simulink model "state_estimator_opt_driftingcar_multibeta"  (R2017a)
settings: Solver=FixedStepAuto  StartTime=0.0  StopTime=inf  FixedStep=1e-3  RelTol=1e-3
InitFcn:
  | state_estimator_opt_driftingcar_multibeta_callback
values from neighbouring files (symbols this model uses):
  acc_integrator_initial_condition = [0,0,0,0.1]    [state_estimator_opt_driftingcar_multibeta_callback.m]
  Den_PDa = [1 0.1111]    [state_estimator_opt_driftingcar_multibeta_callback.m]
  ds_nonzero_threshold = 1e-3    (= 0.001)    [state_estimator_opt_driftingcar_multibeta_callback.m]
  Kp = 500    [state_estimator_opt_driftingcar_multibeta_callback.m]
  Num_PDa = [2.8403 -2.7708]*1e5    [state_estimator_opt_driftingcar_multibeta_callback.m]
  p = 0.1    [state_estimator_opt_driftingcar_multibeta_callback.m]
undefined symbols (not defined in the file or in its folder): DiscIntNeverNeededParam, magnitude
libraries: robotlib x15, simulink x5, dspsigops x4, sharedtransform x1
settings Model: Creator=bascetta  LastModifiedBy=marco
settings OptimizationCC: PassReuseOutputArgsAs=Individual arguments  MaxStackSize=64
settings DebuggingCC: ParameterTunabilityLossMsg=error
settings HardwareCC: ProdBitPerPointer=32  ProdBitPerSizeT=32  ProdBitPerPtrDiffT=32  ProdLargestAtomicFloat=None  ProdIntDivRoundTo=Undefined  ProdEndianess=Unspecified  ProdWordSize=32  ProdHWDeviceType=Generic->Unspecified (assume 32-bit Generic)
settings SFSimCC: MATLABDynamicMemAlloc=off
settings RTWCC: SystemTargetFile=ert.tlc  HardwareBoard=Robot Operating System (ROS)  TLCOptions="-aInlineSetEventsForThisBaseRateFcn=TLC_FALSE -aSuppressMultiTaskScheduler=TLC_FALSE  -aRateBasedStepFcn=0"  TemplateMakefile=ert_default_tmf  Description=Embedded Coder  GenerateReport=on  Toolchain=Catkin  IncludeHyperlinkInReport=on  LaunchReport=on  TargetLang=C++  GenerateTraceInfo=on  GenerateTraceReport=on  GenerateTraceReportSl=on  GenerateTraceReportSf=on  GenerateTraceReportEml=on
settings CodeAppCC: ForceParamTrailComments=on  IgnoreCustomStorageClasses=off  OperatorAnnotations=on  SimulinkDataObjDesc=on  SFDataObjDesc=on  MATLABFcnDesc=on  InsertBlockDesc=on  MATLABSourceComments=on
settings ConfigComp: CovScope=ReferencedModels  CovIncludeTopModel=off

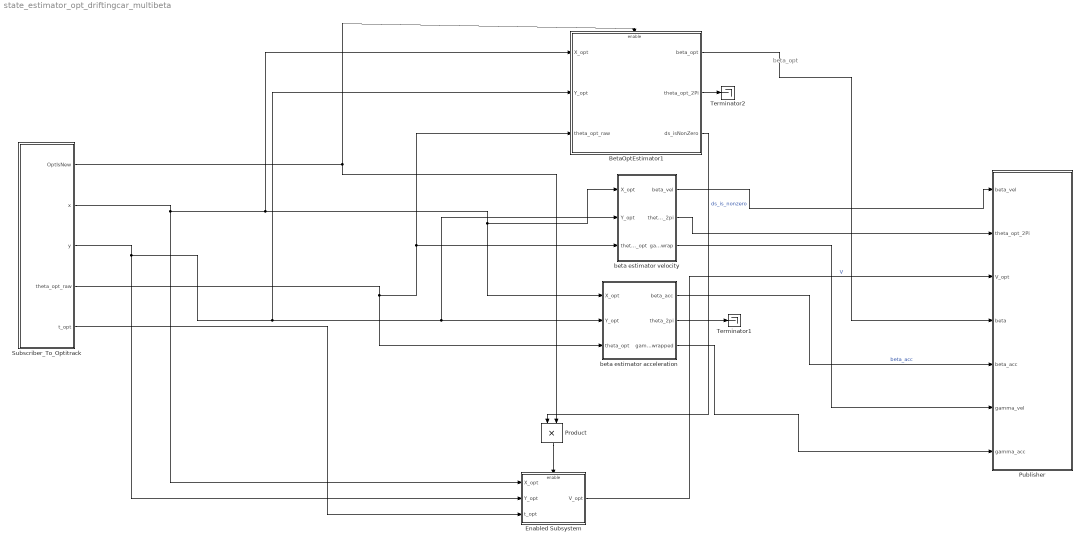
== system state_estimator_opt_driftingcar_multibeta ==
  note: beta_opt
  BetaOptEstimator1 : Subsystem
  Enabled Subsystem : Subsystem  TreatAsAtomicUnit=on
  Product : Product
  Publisher : Subsystem
  Subscriber_To_Optitrack : Subsystem
  Terminator1 : Terminator
  Terminator2 : Terminator
  beta estimator acceleration : Subsystem
  beta estimator velocity : Subsystem
  wires:
  Subscriber_To_Optitrack/4(theta_opt_raw) -> beta estimator acceleration/3(theta_opt), BetaOptEstimator1/3(theta_opt_raw), beta estimator velocity/3(theta_opt)
  Product/1 -> Enabled Subsystem/Enable
  Subscriber_To_Optitrack/5(t_opt) -> Enabled Subsystem/3(t_opt)
  Enabled Subsystem/1(V_opt) -> Publisher/3(V_opt)  "V"
  BetaOptEstimator1/1(beta_opt) -> Publisher/4(beta)
  BetaOptEstimator1/2(theta_opt_2Pi) -> Terminator2/1
  beta estimator velocity/1(beta_vel) -> Publisher/1(beta_vel)
  beta estimator velocity/2(theta_2pi) -> Publisher/2(theta_opt_2Pi)
  beta estimator acceleration/2(theta_2pi) -> Terminator1/1
  beta estimator acceleration/1(beta_acc) -> Publisher/5(beta_acc)  "beta_acc"
  beta estimator acceleration/3(gamma_acc_unwrapped) -> Publisher/7(gamma_acc)
  beta estimator velocity/3(gamma_vel_unwrap) -> Publisher/6(gamma_vel)
  BetaOptEstimator1/3(ds_isNonZero) -> Product/1  "ds_is_nonzero"
  Subscriber_To_Optitrack/3(y) -> Enabled Subsystem/2(Y_opt), BetaOptEstimator1/2(Y_opt), beta estimator velocity/2(Y_opt), beta estimator acceleration/2(Y_opt)
  Subscriber_To_Optitrack/2(x) -> Enabled Subsystem/1(X_opt), BetaOptEstimator1/1(X_opt), beta estimator velocity/1(X_opt), beta estimator acceleration/1(X_opt)
  Subscriber_To_Optitrack/1(OptIsNew) -> Product/2, BetaOptEstimator1/Enable

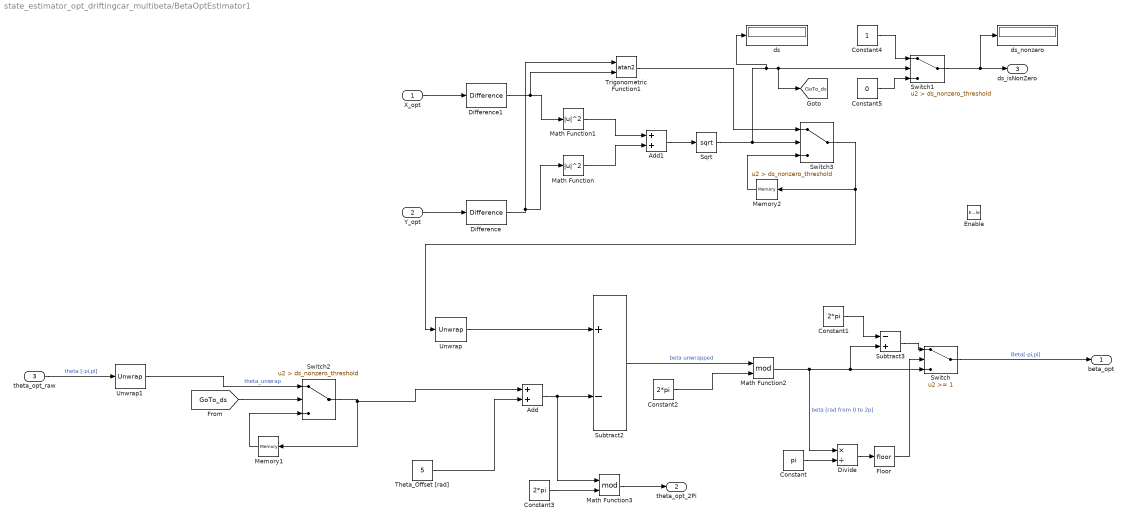
== system state_estimator_opt_driftingcar_multibeta/BetaOptEstimator1 ==
  X_opt : Inport
  Y_opt : Inport  Port=2
  theta_opt_raw : Inport  Port=3
  Enable : EnablePort
  Add : Sum
  Add1 : Sum
  Constant : Constant  Value=pi
  Constant1 : Constant  Value=2*pi
  Constant2 : Constant  Value=2*pi
  Constant3 : Constant  Value=2*pi
  Constant4 : Constant
  Constant5 : Constant  Value=0
  Difference : simulink/Discrete/Difference  ICPrevInput=0.0  OutMin=[]  OutMax=[]  OutDataType=fixdt(1, 16)  OutScaling=2^-10  DoSatur=off
  Difference1 : simulink/Discrete/Difference  ICPrevInput=0.0  OutMin=[]  OutMax=[]  OutDataType=fixdt(1, 16)  OutScaling=2^-10  DoSatur=off
  Divide : Product  Inputs=*/
  Floor : Rounding
  Math Function : Math  Operator=magnitude^2  SaturateOnIntegerOverflow=on
  Math Function1 : Math  Operator=magnitude^2  SaturateOnIntegerOverflow=on
  Math Function2 : Math  Operator=mod  SaturateOnIntegerOverflow=on
  Math Function3 : Math  Operator=mod  SaturateOnIntegerOverflow=on
  Memory1 : Memory
  Memory2 : Memory
  Sqrt : Sqrt  SaturateOnIntegerOverflow=on
  Subtract2 : Sum  Inputs=+-
  Subtract3 : Sum  Inputs=-+
  Switch : Switch  Threshold=1
  Switch1 : Switch  Criteria=u2 > Threshold  Threshold=ds_nonzero_threshold
  Switch2 : Switch  Criteria=u2 > Threshold  Threshold=ds_nonzero_threshold
  Switch3 : Switch  Criteria=u2 > Threshold  Threshold=ds_nonzero_threshold
  Theta_Offset [rad] : Constant  Value=5
  Trigonometric Function1 : Trigonometry  Operator=atan2
  Unwrap : dspsigops/Unwrap  tol=pi  InputProcessing=Columns as channels (frame based)  running=off
  Unwrap1 : dspsigops/Unwrap  tol=pi  InputProcessing=Columns as channels (frame based)  running=off
  ds : Display
  ds_nonzero : Display
  beta_opt : Outport
  theta_opt_2Pi : Outport  Port=2
  ds_isNonZero : Outport  Port=3
  tag scope: GoTo_ds=global
  wires:
  X_opt/1 -> Difference1/1
  Constant/1 -> Divide/2
  Divide/1 -> Floor/1
  Constant2/1 -> Math Function2/2
  Subtract3/1 -> Switch/1
  Subtract2/1 -> Math Function2/1  "beta unwrapped"
  Unwrap/1 -> Subtract2/1
  Math Function2/1 -> Divide/1, Subtract3/2, Switch/3  "beta [rad from 0 to 2p]"
  Floor/1 -> Switch/2
  Switch/1 -> beta_opt/1  "Beta[-pi,pi]"
  theta_opt_raw/1 -> Unwrap1/1  "theta [-pi,pi]"
  Theta_Offset [rad]/1 -> Add/2
  Add/1 -> Math Function3/1, Subtract2/2
  Constant1/1 -> Subtract3/1
  Y_opt/1 -> Difference/1
  Math Function1/1 -> Add1/1
  Difference/1 -> Trigonometric Function1/1, Math Function/1
  Switch3/1 -> Unwrap/1, Memory2/1
  Difference1/1 -> Trigonometric Function1/2, Math Function1/1
  Add1/1 -> Sqrt/1
  Math Function/1 -> Add1/2
  Memory2/1 -> Switch3/3
  Trigonometric Function1/1 -> Switch3/1
  Constant3/1 -> Math Function3/2
  Math Function3/1 -> theta_opt_2Pi/1
  Constant5/1 -> Switch1/3
  Constant4/1 -> Switch1/1
  Switch1/1 -> ds_nonzero/1, ds_isNonZero/1
  Sqrt/1 -> ds/1, [GoTo_ds], Switch1/2, Switch3/2
  Memory1/1 -> Switch2/3
  Switch2/1 -> Add/1, Memory1/1
  Unwrap1/1 -> Switch2/1  "theta_unwrap"
  [GoTo_ds] -> Switch2/2

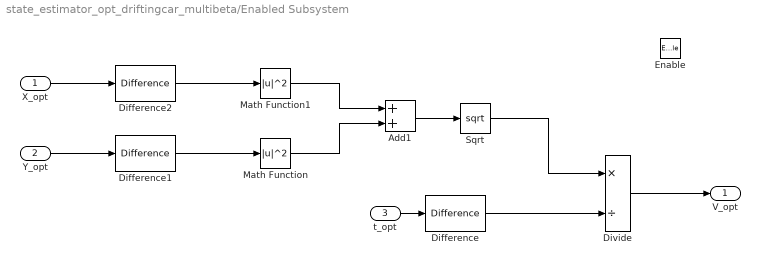
== system state_estimator_opt_driftingcar_multibeta/Enabled Subsystem ==
  X_opt : Inport
  Y_opt : Inport  Port=2
  t_opt : Inport  Port=3
  Enable : EnablePort
  Add1 : Sum
  Difference : simulink/Discrete/Difference  ICPrevInput=0.0  OutMin=[]  OutMax=[]  OutDataType=fixdt(1, 16)  OutScaling=2^-10  DoSatur=off
  Difference1 : simulink/Discrete/Difference  ICPrevInput=0.0  OutMin=[]  OutMax=[]  OutDataType=fixdt(1, 16)  OutScaling=2^-10  DoSatur=off
  Difference2 : simulink/Discrete/Difference  ICPrevInput=0.0  OutMin=[]  OutMax=[]  OutDataType=fixdt(1, 16)  OutScaling=2^-10  DoSatur=off
  Divide : Product  Inputs=*/
  Math Function : Math  Operator=magnitude^2  SaturateOnIntegerOverflow=on
  Math Function1 : Math  Operator=magnitude^2  SaturateOnIntegerOverflow=on
  Sqrt : Sqrt  SaturateOnIntegerOverflow=on
  V_opt : Outport
  wires:
  t_opt/1 -> Difference/1
  Divide/1 -> V_opt/1
  Difference/1 -> Divide/2
  Difference2/1 -> Math Function1/1
  Math Function/1 -> Add1/2
  Difference1/1 -> Math Function/1
  Sqrt/1 -> Divide/1
  Y_opt/1 -> Difference1/1
  Math Function1/1 -> Add1/1
  Add1/1 -> Sqrt/1
  X_opt/1 -> Difference2/1

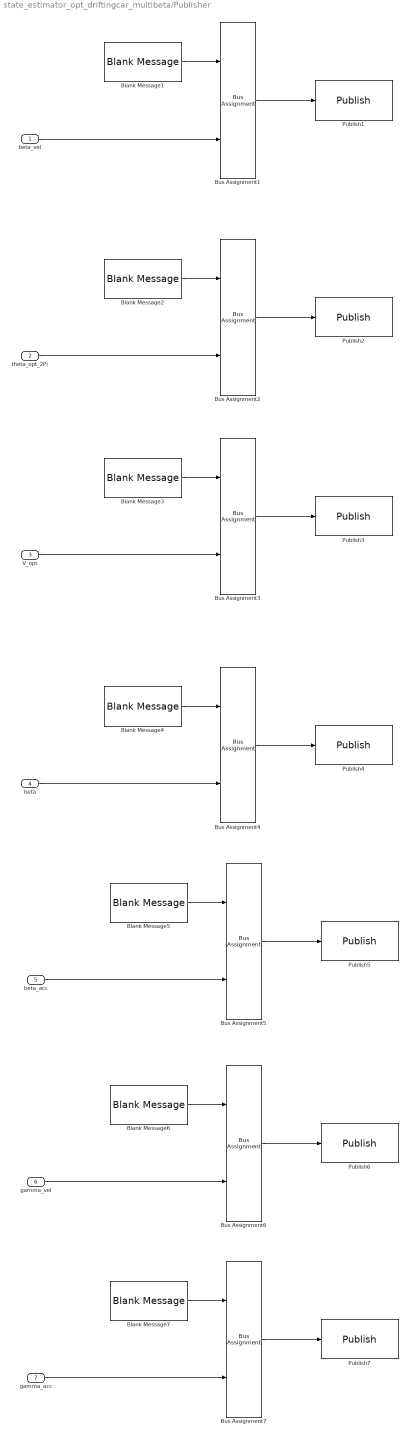
== system state_estimator_opt_driftingcar_multibeta/Publisher ==
  beta_vel : Inport
  theta_opt_2Pi : Inport  Port=2
  V_opt : Inport  Port=3
  beta : Inport  Port=4
  beta_acc : Inport  Port=5
  gamma_vel : Inport  Port=6
  gamma_acc : Inport  Port=7
  Blank Message{1..7} (7 alike) : robotlib/Blank Message  SourceLibraryInfo=This block requires Robotics System Toolbox  messageType=std_msgs/Float64  SampleTime=inf
      settings: SourceProductBaseCode=RO
  Bus Assignment{1..7} (7 alike) : BusAssignment  AssignedSignals=Data
  Publish1 : robotlib/Publish  SourceLibraryInfo=This block requires Robotics System Toolbox  topicSource=Specify your own  topic=/state_estimator_opt_beta_vel  messageType=std_msgs/Float64  messageQueueLength=1
      settings: SourceProductBaseCode=RO
  Publish2 : robotlib/Publish  SourceLibraryInfo=This block requires Robotics System Toolbox  topicSource=Specify your own  topic=/state_estimator_opt_theta  messageType=std_msgs/Float64  messageQueueLength=1
      settings: SourceProductBaseCode=RO
  Publish3 : robotlib/Publish  SourceLibraryInfo=This block requires Robotics System Toolbox  topicSource=Specify your own  topic=/state_estimator_opt_V  messageType=std_msgs/Float64  messageQueueLength=1
      settings: SourceProductBaseCode=RO
  Publish4 : robotlib/Publish  SourceLibraryInfo=This block requires Robotics System Toolbox  topicSource=Specify your own  topic=/state_estimator_opt_beta  messageType=std_msgs/Float64  messageQueueLength=1
      settings: SourceProductBaseCode=RO
  Publish5 : robotlib/Publish  SourceLibraryInfo=This block requires Robotics System Toolbox  topicSource=Specify your own  topic=/state_estimator_opt_beta_acc  messageType=std_msgs/Float64  messageQueueLength=1
      settings: SourceProductBaseCode=RO
  Publish6 : robotlib/Publish  SourceLibraryInfo=This block requires Robotics System Toolbox  topicSource=Specify your own  topic=/state_estimator_opt_gamma_vel  messageType=std_msgs/Float64  messageQueueLength=1
      settings: SourceProductBaseCode=RO
  Publish7 : robotlib/Publish  SourceLibraryInfo=This block requires Robotics System Toolbox  topicSource=Specify your own  topic=/state_estimator_opt_gamma_acc  messageType=std_msgs/Float64  messageQueueLength=1
      settings: SourceProductBaseCode=RO
  wires:
  beta_vel/1 -> Bus Assignment1/2
  Blank Message1/1 -> Bus Assignment1/1
  Bus Assignment1/1 -> Publish1/1
  theta_opt_2Pi/1 -> Bus Assignment2/2
  Blank Message2/1 -> Bus Assignment2/1
  Bus Assignment2/1 -> Publish2/1
  V_opt/1 -> Bus Assignment3/2
  Blank Message3/1 -> Bus Assignment3/1
  Bus Assignment3/1 -> Publish3/1
  beta/1 -> Bus Assignment4/2
  Bus Assignment4/1 -> Publish4/1
  Blank Message4/1 -> Bus Assignment4/1
  Bus Assignment5/1 -> Publish5/1
  beta_acc/1 -> Bus Assignment5/2
  Blank Message5/1 -> Bus Assignment5/1
  Bus Assignment6/1 -> Publish6/1
  gamma_vel/1 -> Bus Assignment6/2
  Blank Message6/1 -> Bus Assignment6/1
  Bus Assignment7/1 -> Publish7/1
  gamma_acc/1 -> Bus Assignment7/2
  Blank Message7/1 -> Bus Assignment7/1

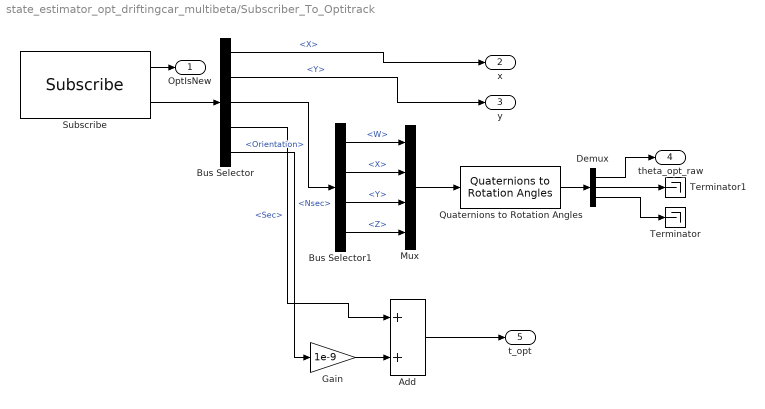
== system state_estimator_opt_driftingcar_multibeta/Subscriber_To_Optitrack ==
  Add : Sum
  Bus Selector : BusSelector  OutputSignals=Pose.Position.X,Pose.Position.Y,Pose.Orientation,Header.Stamp.Sec,Header.Stamp.Nsec
  Bus Selector1 : BusSelector  OutputSignals=W,X,Y,Z
  Demux : Demux  Outputs=3
  Gain : Gain  Gain=1e-9
  Mux : Mux
  Quaternions to Rotation Angles : sharedtransform/Quaternions to Rotation Angles  rotationOrder=ZYX
  Subscribe : robotlib/Subscribe  SourceLibraryInfo=This block requires Robotics System Toolbox  topicSource=Specify your own  topic=/car/pose  messageType=geometry_msgs/PoseStamped  sampleTime=-1  messageQueueLength=1
      settings: SourceProductBaseCode=RO
  Terminator : Terminator
  Terminator1 : Terminator
  OptIsNew : Outport
  x : Outport  Port=2
  y : Outport  Port=3
  theta_opt_raw : Outport  Port=4
  t_opt : Outport  Port=5
  wires:
  Subscribe/2 -> Bus Selector/1
  Subscribe/1 -> OptIsNew/1
  Bus Selector/1 -> x/1  "<X>"
  Bus Selector/2 -> y/1  "<Y>"
  Quaternions to Rotation Angles/1 -> Demux/1
  Demux/3 -> Terminator/1
  Demux/2 -> Terminator1/1
  Demux/1 -> theta_opt_raw/1
  Mux/1 -> Quaternions to Rotation Angles/1
  Bus Selector/3 -> Bus Selector1/1  "<Orientation>"
  Bus Selector1/1 -> Mux/1  "<W>"
  Bus Selector1/2 -> Mux/2  "<X>"
  Bus Selector1/3 -> Mux/3  "<Y>"
  Bus Selector1/4 -> Mux/4  "<Z>"
  Gain/1 -> Add/2
  Bus Selector/5 -> Gain/1  "<Nsec>"
  Bus Selector/4 -> Add/1  "<Sec>"
  Add/1 -> t_opt/1

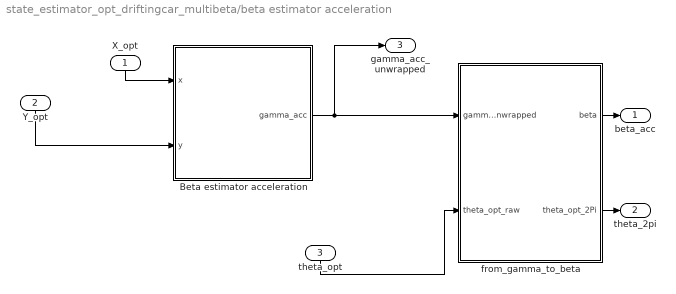
== system state_estimator_opt_driftingcar_multibeta/beta estimator acceleration ==
  X_opt : Inport
  Y_opt : Inport  Port=2
  theta_opt : Inport  Port=3
  Beta estimator acceleration : Subsystem
  from_gamma_to_beta : Subsystem
  beta_acc : Outport
  theta_2pi : Outport  Port=2
  gamma_acc_unwrapped : Outport  Port=3
  wires:
  from_gamma_to_beta/1(beta) -> beta_acc/1
  X_opt/1 -> Beta estimator acceleration/1(x)
  Y_opt/1 -> Beta estimator acceleration/2(y)
  Beta estimator acceleration/1(gamma_acc) -> gamma_acc_unwrapped/1, from_gamma_to_beta/1(gamma_unwrapped)
  from_gamma_to_beta/2(theta_opt_2Pi) -> theta_2pi/1
  theta_opt/1 -> from_gamma_to_beta/2(theta_opt_raw)

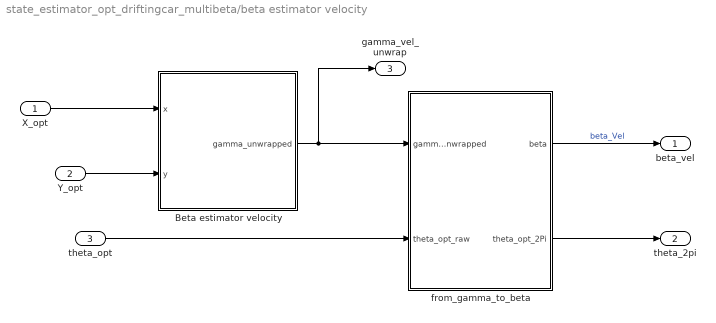
== system state_estimator_opt_driftingcar_multibeta/beta estimator velocity ==
  X_opt : Inport
  Y_opt : Inport  Port=2
  theta_opt : Inport  Port=3
  Beta estimator velocity : Subsystem
  from_gamma_to_beta : Subsystem
  beta_vel : Outport
  theta_2pi : Outport  Port=2
  gamma_vel_unwrap : Outport  Port=3
  wires:
  from_gamma_to_beta/2(theta_opt_2Pi) -> theta_2pi/1
  Beta estimator velocity/1(gamma_unwrapped) -> gamma_vel_unwrap/1, from_gamma_to_beta/1(gamma_unwrapped)
  X_opt/1 -> Beta estimator velocity/1(x)
  theta_opt/1 -> from_gamma_to_beta/2(theta_opt_raw)
  Y_opt/1 -> Beta estimator velocity/2(y)
  from_gamma_to_beta/1(beta) -> beta_vel/1  "beta_Vel"

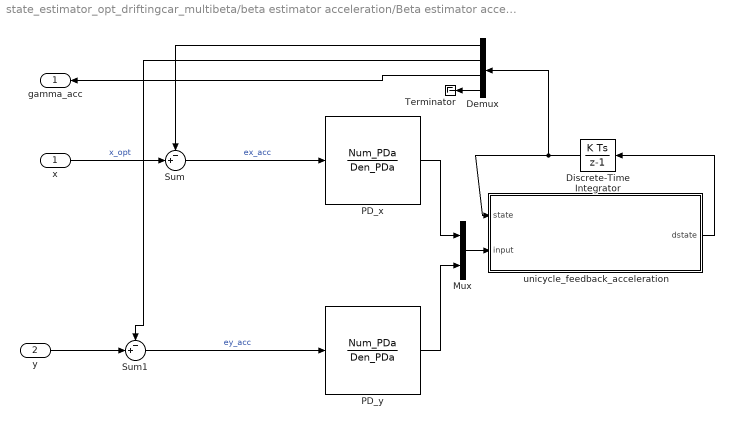
== system state_estimator_opt_driftingcar_multibeta/beta estimator acceleration/Beta estimator acceleration ==
  x : Inport
  y : Inport  Port=2
  Demux : Demux
  Discrete-Time Integrator : DiscreteIntegrator  InitialCondition=acc_integrator_initial_condition  InitialConditionSetting=State (most efficient)  SampleTime=1e-3  ICPrevOutput=DiscIntNeverNeededParam  ICPrevScaledInput=DiscIntNeverNeededParam
  Mux : Mux  Inputs=2
  PD_x : DiscreteTransferFcn  Numerator=Num_PDa  Denominator=Den_PDa  a0EqualsOne=on
  PD_y : DiscreteTransferFcn  Numerator=Num_PDa  Denominator=Den_PDa  a0EqualsOne=on
  Sum : Sum  Inputs=-+|
  Sum1 : Sum  Inputs=-+|
  Terminator : Terminator
  unicycle_feedback_acceleration : MATLAB Function  TreatAsAtomicUnit=on
  gamma_acc : Outport
  wires:
  unicycle_feedback_acceleration/1(dstate) -> Discrete-Time Integrator/1
  Mux/1 -> unicycle_feedback_acceleration/2(input)
  Demux/1 -> Sum/1
  PD_x/1 -> Mux/1
  y/1 -> Sum1/2
  Demux/3 -> gamma_acc/1
  Demux/2 -> Sum1/1
  x/1 -> Sum/2  "x_opt"
  PD_y/1 -> Mux/2
  Discrete-Time Integrator/1 -> Demux/1, unicycle_feedback_acceleration/1(state)
  Demux/4 -> Terminator/1
  Sum1/1 -> PD_y/1  "ey_acc"
  Sum/1 -> PD_x/1  "ex_acc"

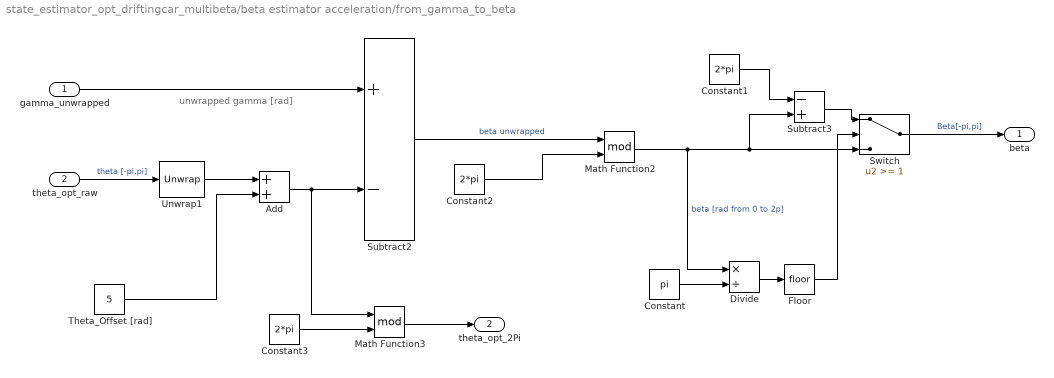
== system state_estimator_opt_driftingcar_multibeta/beta estimator acceleration/from_gamma_to_beta ==
  note: unwrapped gamma [rad]
  gamma_unwrapped : Inport
  theta_opt_raw : Inport  Port=2
  Add : Sum
  Constant : Constant  Value=pi
  Constant1 : Constant  Value=2*pi
  Constant2 : Constant  Value=2*pi
  Constant3 : Constant  Value=2*pi
  Divide : Product  Inputs=*/
  Floor : Rounding
  Math Function2 : Math  Operator=mod  SaturateOnIntegerOverflow=on
  Math Function3 : Math  Operator=mod  SaturateOnIntegerOverflow=on
  Subtract2 : Sum  Inputs=+-
  Subtract3 : Sum  Inputs=-+
  Switch : Switch  Threshold=1
  Theta_Offset [rad] : Constant  Value=5
  Unwrap1 : dspsigops/Unwrap  tol=pi  InputProcessing=Columns as channels (frame based)  running=off
  beta : Outport
  theta_opt_2Pi : Outport  Port=2
  wires:
  Math Function3/1 -> theta_opt_2Pi/1
  theta_opt_raw/1 -> Unwrap1/1  "theta [-pi,pi]"
  Theta_Offset [rad]/1 -> Add/2
  gamma_unwrapped/1 -> Subtract2/1
  Constant3/1 -> Math Function3/2
  Constant/1 -> Divide/2
  Constant1/1 -> Subtract3/1
  Subtract2/1 -> Math Function2/1  "beta unwrapped"
  Divide/1 -> Floor/1
  Subtract3/1 -> Switch/1
  Switch/1 -> beta/1  "Beta[-pi,pi]"
  Add/1 -> Math Function3/1, Subtract2/2
  Math Function2/1 -> Divide/1, Subtract3/2, Switch/3  "beta [rad from 0 to 2p]"
  Unwrap1/1 -> Add/1
  Floor/1 -> Switch/2
  Constant2/1 -> Math Function2/2

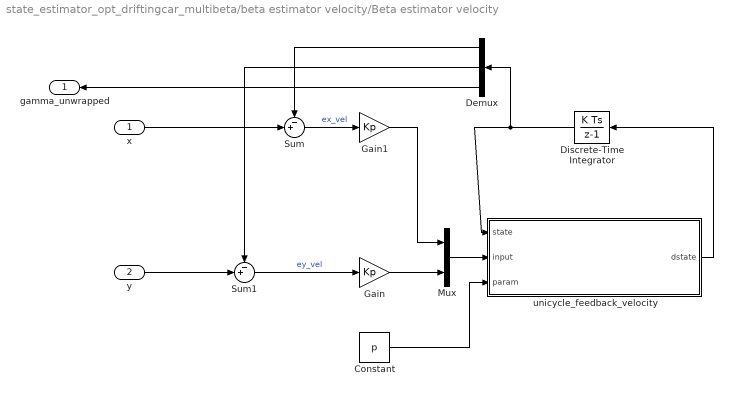
== system state_estimator_opt_driftingcar_multibeta/beta estimator velocity/Beta estimator velocity ==
  x : Inport
  y : Inport  Port=2
  Constant : Constant  Value=p
  Demux : Demux  Outputs=3
  Discrete-Time Integrator : DiscreteIntegrator  InitialConditionSetting=State (most efficient)  SampleTime=0.001  ICPrevOutput=DiscIntNeverNeededParam  ICPrevScaledInput=DiscIntNeverNeededParam
  Gain : Gain  Gain=Kp
  Gain1 : Gain  Gain=Kp
  Mux : Mux  Inputs=2
  Sum : Sum  Inputs=-+|
  Sum1 : Sum  Inputs=-+|
  unicycle_feedback_velocity : MATLAB Function  TreatAsAtomicUnit=on
  gamma_unwrapped : Outport
  wires:
  Demux/3 -> gamma_unwrapped/1
  y/1 -> Sum1/2
  Demux/1 -> Sum/1
  Sum1/1 -> Gain/1  "ey_vel"
  Gain/1 -> Mux/2
  Gain1/1 -> Mux/1
  Mux/1 -> unicycle_feedback_velocity/2(input)
  Constant/1 -> unicycle_feedback_velocity/3(param)
  Sum/1 -> Gain1/1  "ex_vel"
  Demux/2 -> Sum1/1
  x/1 -> Sum/2
  unicycle_feedback_velocity/1(dstate) -> Discrete-Time Integrator/1
  Discrete-Time Integrator/1 -> Demux/1, unicycle_feedback_velocity/1(state)

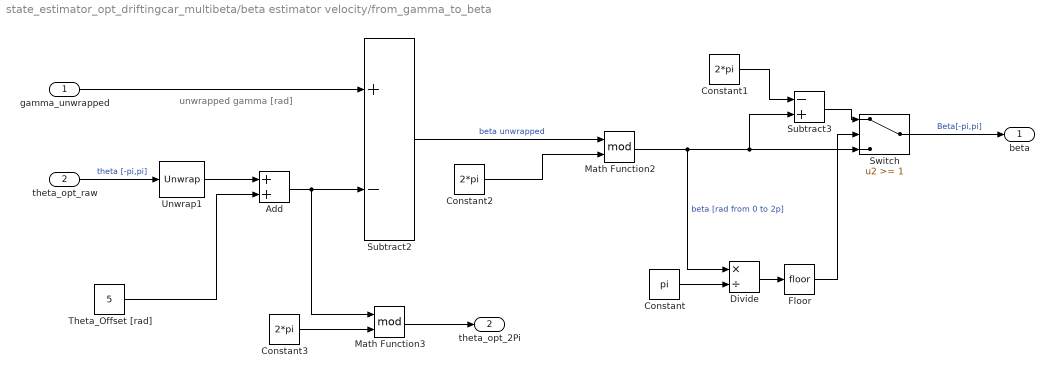
== system state_estimator_opt_driftingcar_multibeta/beta estimator velocity/from_gamma_to_beta ==
  note: unwrapped gamma [rad]
  gamma_unwrapped : Inport
  theta_opt_raw : Inport  Port=2
  Add : Sum
  Constant : Constant  Value=pi
  Constant1 : Constant  Value=2*pi
  Constant2 : Constant  Value=2*pi
  Constant3 : Constant  Value=2*pi
  Divide : Product  Inputs=*/
  Floor : Rounding
  Math Function2 : Math  Operator=mod  SaturateOnIntegerOverflow=on
  Math Function3 : Math  Operator=mod  SaturateOnIntegerOverflow=on
  Subtract2 : Sum  Inputs=+-
  Subtract3 : Sum  Inputs=-+
  Switch : Switch  Threshold=1
  Theta_Offset [rad] : Constant  Value=5
  Unwrap1 : dspsigops/Unwrap  tol=pi  InputProcessing=Columns as channels (frame based)  running=off
  beta : Outport
  theta_opt_2Pi : Outport  Port=2
  wires:
  Math Function3/1 -> theta_opt_2Pi/1
  theta_opt_raw/1 -> Unwrap1/1  "theta [-pi,pi]"
  Theta_Offset [rad]/1 -> Add/2
  gamma_unwrapped/1 -> Subtract2/1
  Constant3/1 -> Math Function3/2
  Constant/1 -> Divide/2
  Constant1/1 -> Subtract3/1
  Subtract2/1 -> Math Function2/1  "beta unwrapped"
  Divide/1 -> Floor/1
  Subtract3/1 -> Switch/1
  Switch/1 -> beta/1  "Beta[-pi,pi]"
  Add/1 -> Math Function3/1, Subtract2/2
  Math Function2/1 -> Divide/1, Subtract3/2, Switch/3  "beta [rad from 0 to 2p]"
  Unwrap1/1 -> Add/1
  Floor/1 -> Switch/2
  Constant2/1 -> Math Function2/2

== matlab function state_estimator_opt_driftingcar_multibeta/beta estimator velocity/Beta estimator velocity/unicycle_feedback_velocity ==
  data: state input size=3; dstate output size=3; input input size=2; param input size=1
function dstate = unicycle_feedback_velocity(state,input,param)

% State and input variables
x     = state(1);
y     = state(2);
gamma = state(3); % theta+beta

vxp   = input(1);
vyp   = input(2);

% Parameters
p = param(1);

% Model equations
dstate = zeros(3,1);
dstate(1) = vxp*cos(gamma)^2+vyp*sin(gamma)*cos(gamma);
dstate(2) = vxp*sin(gamma)*cos(gamma)+vyp*sin(gamma)^2;
dstate(3) = (vyp*cos(gamma)-vxp*sin(gamma))/p;

== matlab function state_estimator_opt_driftingcar_multibeta/beta estimator acceleration/Beta estimator acceleration/unicycle_feedback_acceleration ==
  data: state input size=4; dstate output size=4; input input size=2
function dstate = unicycle_feedback_acceleration(state,input)

% State and input variables
x     = state(1); %[m]
y     = state(2); %[m]
gamma = state(3); % theta+beta [rad]
v     = state(4); %[m/s]

ax    = input(1); %[m/s^2]
ay    = input(2); %[m/s^2]

% Model equations
dstate = zeros(4,1);
dstate(1) = v*cos(gamma); %dx/dt
dstate(2) = v*sin(gamma); %dy/dt
dstate(3) = (ay*cos(gamma)-ax*sin(gamma))/v; %d(gamma)/dt
dstate(4) = ax*cos(gamma)+ay*sin(gamma); %dv/dt
